simulink model "dvr_final"  (R2017b)
settings: Solver=ode45  StartTime=0.0  StopTime=1  RelTol=1e-3  EnableMultiTasking=on
undefined symbols (not defined in the file): D1, Delta, Ts
libraries: powerlib x28, powerlib_extras x19
settings Model: Creator=PRAVAT  LastModifiedBy=HP
settings DataIOCC: LimitDataPoints=on  SaveFormat=Array  SignalLoggingSaveFormat=ModelDataLogs
settings OptimizationCC: ExpressionDepthLimit=2147483647  LifeSpan=inf
settings DebuggingCC: UnderspecifiedInitializationDetection=Classic  MergeDetectMultiDrivingBlocksExec=none  SolverPrmCheckMsg=warning  FcnCallInpInsideContextMsg=warning  StateNameClashWarn=warning  StrictBusMsg=Warning  SFUnexpectedBacktrackingDiag=warning  SFNoUnconditionalDefaultTransitionDiag=warning  SFExecutionAtInitializationDiag=none
settings HardwareCC: ProdBitPerPointer=32  ProdBitPerSizeT=32  ProdBitPerPtrDiffT=32  ProdLargestAtomicFloat=None  ProdIntDivRoundTo=Undefined  ProdEndianess=Unspecified  ProdWordSize=32  ProdHWDeviceType=32-bit Generic
settings ModelReferenceCC: PropagateSignalLabelsOutOfModel=off
settings CodeAppCC: StateflowObjectComments=on
settings GRTTargetCC: TargetLangStandard=C89/C90 (ANSI)  CombineOutputUpdateFcns=off  GRTInterface=on
settings ConfigComp: CovMetricSettings=dw  CovHtmlReporting=on  CovSaveCumulativeToWorkspaceVar=on  CovSaveSingleToWorkspaceVar=on  CovExternalEMLEnable=off

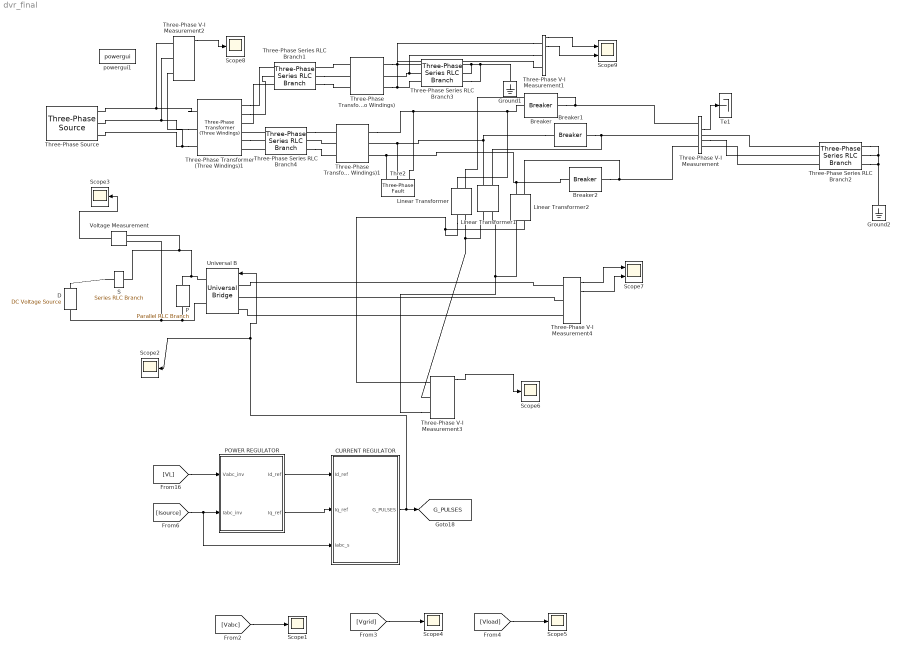
== system dvr_final ==
  Breaker : powerlib/Elements/Breaker  InitialState=1  SwitchingTimes=[0.4 0.6]  External=off  BreakerResistance=0.01  SnubberResistance=1e6  SnubberCapacitance=inf  Measurements=None  MoreParameters=off  NoBreakLoop=off
      settings: SourceProductName=Simscape Power Systems
  Breaker1 : powerlib/Elements/Breaker  InitialState=1  SwitchingTimes=[0.4 0.6]  External=off  BreakerResistance=0.01  SnubberResistance=1e6  SnubberCapacitance=inf  Measurements=None  MoreParameters=off  NoBreakLoop=off
      settings: SourceProductName=Simscape Power Systems
  Breaker2 : powerlib/Elements/Breaker  InitialState=1  SwitchingTimes=[0.4 0.6]  External=off  BreakerResistance=0.01  SnubberResistance=1e6  SnubberCapacitance=inf  Measurements=None  MoreParameters=off  NoBreakLoop=off
      settings: SourceProductName=Simscape Power Systems
  CURRENT REGULATOR : Subsystem
  D : powerlib/Electrical Sources/DC Voltage Source  Amplitude=5e3  Measurements=None
  Ground1 : powerlib/Elements/Ground  LConnTagsString=a
  Ground2 : powerlib/Elements/Ground  LConnTagsString=a
  Linear Transformer : powerlib/Elements/Linear Transformer  UNITS=pu  NominalPower=[ 250e6 50 ]  winding1="[11e3  0.002  0.08 ]"  winding2="[9e3  0.002  0.08 ]"  ThreeWindings=off  winding3=[ 60e3 0.005 0.02 ]  RmLm=[ 500 500 ]  Measurements=None  DataType=off
  Linear Transformer1 : powerlib/Elements/Linear Transformer  UNITS=pu  NominalPower=[ 250e6 50 ]  winding1="[11e3  0.002  0.08 ]"  winding2="[9e3  0.002  0.08 ]"  ThreeWindings=off  winding3=[ 60e3 0.005 0.02 ]  RmLm=[ 500 500 ]  Measurements=None  DataType=off
  Linear Transformer2 : powerlib/Elements/Linear Transformer  UNITS=pu  NominalPower=[ 250e6 50 ]  winding1="[11e3  0.002  0.08 ]"  winding2="[9e3  0.002  0.08 ]"  ThreeWindings=off  winding3=[ 60e3 0.005 0.02 ]  RmLm=[ 500 500 ]  Measurements=None  DataType=off
  P : powerlib/Elements/Parallel RLC Branch  LConnTagsString=a  RConnTagsString=__new0  BranchType=C  Resistance=[]  Inductance=[]  SetiL0=off  InitialCurrent=0  Capacitance=750e-6  Setx0=off  InitialVoltage=0  Measurements=Branch voltage and current
  POWER REGULATOR : Subsystem
  S : powerlib/Elements/Series RLC Branch  LConnTagsString=__new0  RConnTagsString=__new0  BranchType=R  Resistance=10  Inductance=1e-3  SetiL0=off  InitialCurrent=0  Capacitance=1e-6  Setx0=off  InitialVoltage=0  Measurements=None
  Scope{1..6,8} (7 alike) : Scope
  Scope7 : Scope  NumInputPorts=2
  Scope9 : Scope  NumInputPorts=2
  Te1 : Terminator
  Thre2 : powerlib/Elements/Three-Phase Fault  InitialStates=0  FaultA=on  FaultB=on  FaultC=on  GroundFault=on  SwitchTimes=[ 0.4 0.6]  External=off  SwitchStatus=NaN  FaultResistance=0.66  GroundResistance=0.4  SnubberResistance=1e6  SnubberCapacitance=inf  Measurements=None
  Three-Phase Series RLC Branch1 : powerlib/Elements/Three-Phase Series RLC Branch  LConnTagsString=A|B|C  RConnTagsString=A|B|C  BranchType=RL  Resistance=.05  Inductance=0.4806  Capacitance=1e-6  Measurements=None
  Three-Phase Series RLC Branch2 : powerlib/Elements/Three-Phase Series RLC Branch  LConnTagsString=A|B|C  RConnTagsString=A|B|C  BranchType=RL  Resistance=0.1  Inductance=.1926  Capacitance=1e-6  Measurements=Branch voltages
  Three-Phase Series RLC Branch3 : powerlib/Elements/Three-Phase Series RLC Branch  LConnTagsString=A|B|C  RConnTagsString=A|B|C  BranchType=R  Resistance=20  Inductance=1e-3  Capacitance=1e-6  Measurements=None
  Three-Phase Series RLC Branch4 : powerlib/Elements/Three-Phase Series RLC Branch  LConnTagsString=A|B|C  RConnTagsString=A|B|C  BranchType=RL  Resistance=0.001  Inductance=0.005  Capacitance=1e-6  Measurements=None
  Three-Phase Transformer (Three Windings)1 : powerlib/Elements/Three-Phase Transformer (Three Windings)  Winding1Connection=Yg  Winding2Connection=Delta (D1)  Winding3Connection=Delta (D1)  CoreType=Three single-phase transformers  SetSaturation=off  Hysteresis=off  DataFile='hysteresis'  SetInitialFlux=off  Measurements=None  UNITS=pu  NominalPower=[ 100e6 , 50 ]  Winding1=[13e3 , 0.002 , 0.08 ]  Winding2=[115e3 , 0.002 , 0.08 ]  Winding3=[115e3 , 0.002 , 0.08 ]  Rm=500  Lm=500  L0=0.5  Saturation=[ 0,0 ; 0.0024,1.2 ; 1.0,1.52 ]  InitialFluxes=[0.8 -0.8 0.7]  MoreParameters=off  BreakLoop=off  DataType=off  TransfoNumber=0
      settings: SourceProductName=Simscape Power Systems  SourceProductBaseCode=PS
  Three-Phase Transformer (Two Windings) : powerlib/Elements/Three-Phase Transformer (Two Windings)  Winding1Connection=Delta (D1)  Winding2Connection=Yg  CoreType=Three single-phase transformers  SetSaturation=off  Hysteresis=off  DataFile='hysteresis'  SetInitialFlux=off  Measurements=None  UNITS=pu  NominalPower=[ 250e6 , 50 ]  Winding1=[ 115e3 , 0.002 , 0.08 ]  Winding2=[ 11e3 , 0.002 , 0.08 ]  Rm=500  Lm=500  L0=0.5  Saturation=[ 0,0 ; 0.0024,1.2 ; 1.0,1.52 ]  InitialFluxes=[ 0.8 , -0.8 , 0.7 ]  MoreParameters=off  BreakLoop=off  DataType=off  TransfoNumber=0
  Three-Phase Transformer (Two Windings)1 : powerlib/Elements/Three-Phase Transformer (Two Windings)  Winding1Connection=Y  Winding2Connection=Delta (D1)  CoreType=Three single-phase transformers  SetSaturation=off  Hysteresis=off  DataFile='hysteresis'  SetInitialFlux=off  Measurements=None  UNITS=pu  NominalPower=[ 250e6 , 50 ]  Winding1=[ 115e3 , 0.002 , 0.08 ]  Winding2=[ 11e3 , 0.002 , 0.08 ]  Rm=500  Lm=500  L0=0.5  Saturation=[ 0,0 ; 0.0024,1.2 ; 1.0,1.52 ]  InitialFluxes=[ 0.8 , -0.8 , 0.7 ]  MoreParameters=off  BreakLoop=off  DataType=off  TransfoNumber=0
  Three-Phase V-I Measurement : powerlib/Measurements/Three-Phase V-I Measurement  VoltageMeasurement=phase-to-ground  SetLabelV=off  LabelV=Vabc  Vpu=on  VpuLL=off  CurrentMeasurement=yes  SetLabelI=off  LabelI=Iabc  Ipu=on  Pbase=100e6  Vbase=11e3  OutputType=Complex  PhasorSimulation=off  PSBequivalent=0
  Three-Phase V-I Measurement1 : powerlib/Measurements/Three-Phase V-I Measurement  VoltageMeasurement=phase-to-ground  SetLabelV=off  LabelV=Vabc  Vpu=on  VpuLL=off  CurrentMeasurement=yes  SetLabelI=off  LabelI=Iabc  Ipu=on  Pbase=100e6  Vbase=11e3  OutputType=Complex  PhasorSimulation=off  PSBequivalent=0
  Three-Phase V-I Measurement2 : powerlib/Measurements/Three-Phase V-I Measurement  VoltageMeasurement=phase-to-ground  SetLabelV=off  LabelV=Vabc  Vpu=on  VpuLL=off  CurrentMeasurement=yes  SetLabelI=off  LabelI=Iabc  Ipu=on  Pbase=100e6  Vbase=11e3  OutputType=Complex  PhasorSimulation=off  PSBequivalent=0
  Three-Phase V-I Measurement3 : powerlib/Measurements/Three-Phase V-I Measurement  VoltageMeasurement=phase-to-phase  SetLabelV=off  LabelV=Vabc  Vpu=on  VpuLL=off  CurrentMeasurement=yes  SetLabelI=off  LabelI=Iabc  Ipu=on  Pbase=100e6  Vbase=11e3  OutputType=Complex  PhasorSimulation=off  PSBequivalent=0
  Three-Phase V-I Measurement4 : powerlib/Measurements/Three-Phase V-I Measurement  VoltageMeasurement=phase-to-phase  SetLabelV=off  LabelV=Vabc  Vpu=on  VpuLL=off  CurrentMeasurement=yes  SetLabelI=off  LabelI=Iabc  Ipu=on  Pbase=100e6  Vbase=11e3  OutputType=Complex  PhasorSimulation=off  PSBequivalent=0
  Three-Phase Source : powerlib/Electrical Sources/Three-Phase Source  InternalConnection=Yg  VoltagePhases=off  Voltage=13e3  PhaseAngle=0  Voltage_phases=[25e3 25e3 25e3]/sqrt(3)  PhaseAngles_phases=[0 -120 +120]  Frequency=50  NonIdealSource=on  SpecifyImpedance=off  Resistance=0.1  Inductance=0  ShortCircuitLevel=100e6  BaseVoltage=25e3  XRratio=7  BusType=swing  Pref=10e3  Qref=0  Prefabc=[10e3, 10e3, 10e3]  Qrefabc=[0, 0, 0]  Qmin=-inf  Qmax=inf
  Universal B : powerlib/Power Electronics/Universal Bridge  Arms=3  SnubberResistance=1e5  SnubberCapacitance=inf  Device=IGBT / Diodes  Ron=1e-3  Lon=0  ForwardVoltages="[  0  0  ]"  ForwardVoltage=0  GTOparameters=[ 10e-6 , 20e-6 ]  IGBTparameters=[ 1e-6 , 2e-6 ]  Measurements=None  Measurements_2=None  converterType=Rectifier
      link override Uswitch: GotoTag=tp182559
  Voltage Measurement : powerlib/Measurements/Voltage Measurement  PhasorSimulation=off  OutputType=Complex  PSBequivalent=0
  powergui1 : powerlib/powergui  SimulationMode=Discrete  SampleTime=1e-5  frequency=60  Iterations=50  frequencyindice=50  Pbase=100e6  ErrMax=1e-4  UnitsV=kV  UnitsW=MW  buscounter=0  FunctionMessages=off  echomessages=off  EnableUseOfTLC=off  CurrentSourceSwitches=off  DisableSnubberDevices=off  DisableRonSwitches=off  DisableVfSwitches=off  DisplayEquations=off  SolverType=Tustin/Backward Euler (TBE)  Interpol=off  ExternalGateDelay=off  methode=off  Ts=0  x0status=blocks  SPID=off  SwTol=0  HookPort=off  RestoreLinks=warning  ResistiveCurrentMeasurement=off  Frange=[0:2:500]  Ylog=off  Xlog=on  ShowGrid=off  save=off  variable=ZData  structure=0  ZoomFFT=on  StartTime=0.0  cycles=1  DisplayStyle=1  fundamental=60  FreqAxis=off  MaxFrequency=1000  frequencyindicesteady=1  RmsSteady=1  display=off
  tag scope: G_PULSES=global
  wires:
  Voltage Measurement/1 -> Scope3/1
  Three-Phase V-I Measurement3/1 -> Scope6/1
  Three-Phase V-I Measurement4/1 -> Scope7/1
  CURRENT REGULATOR/1(G_PULSES) -> [G_PULSES], Universal B/1, Scope2/1
  POWER REGULATOR/1(Id_ref) -> CURRENT REGULATOR/1(Id_ref)
  POWER REGULATOR/2(Iq_ref) -> CURRENT REGULATOR/2(Iq_ref)
  [VL] -> POWER REGULATOR/1(Vabc_inv)
  [Isource] -> CURRENT REGULATOR/3(Iabc_s), POWER REGULATOR/2(Iabc_inv)
  [Vabc] -> Scope1/1
  [Vgrid] -> Scope4/1
  [Vload] -> Scope5/1
  Three-Phase V-I Measurement2/1 -> Scope8/1
  Three-Phase V-I Measurement/2 -> Te1/1
  Three-Phase V-I Measurement1/1 -> Scope9/1
  Three-Phase V-I Measurement1/2 -> Scope9/2
  Three-Phase V-I Measurement4/2 -> Scope7/2
  connections:
  P/LConn1 -- Universal B/RConn1 -- Voltage Measurement/LConn1 -- S/RConn1
  D/LConn1 -- Voltage Measurement/LConn2 -- Universal B/RConn2 -- P/RConn1
  Three-Phase V-I Measurement3/LConn1 -- Linear Transformer/RConn1 -- Linear Transformer2/RConn2
  Three-Phase V-I Measurement3/LConn2 -- Linear Transformer1/RConn1 -- Linear Transformer/RConn2
  Three-Phase V-I Measurement3/LConn3 -- Linear Transformer2/RConn1 -- Linear Transformer1/RConn2
  Three-Phase V-I Measurement4/LConn2 -- Universal B/LConn2
  Three-Phase V-I Measurement4/LConn1 -- Universal B/LConn1
  Three-Phase V-I Measurement4/LConn3 -- Universal B/LConn3
  S/LConn1 -- D/RConn1
  Three-Phase V-I Measurement1/LConn3 -- Three-Phase Transformer (Two Windings)/RConn3 -- Three-Phase Series RLC Branch3/LConn3
  Three-Phase Transformer (Three Windings)1/LConn2 -- Three-Phase Source/RConn2 -- Three-Phase V-I Measurement2/LConn2
  Breaker/RConn1 -- Linear Transformer/LConn2 -- Three-Phase V-I Measurement/LConn1
  Breaker1/LConn1 -- Linear Transformer1/LConn1 -- Thre2/LConn2 -- Three-Phase Transformer (Two Windings)1/RConn2
  Breaker/LConn1 -- Thre2/LConn1 -- Three-Phase Transformer (Two Windings)1/RConn1 -- Linear Transformer/LConn1
  Three-Phase Series RLC Branch2/RConn1 -- Ground2/LConn1 -- Three-Phase Series RLC Branch2/RConn3 -- Three-Phase Series RLC Branch2/RConn2
  Three-Phase Series RLC Branch3/RConn3 -- Three-Phase Series RLC Branch3/RConn2 -- Three-Phase Series RLC Branch3/RConn1 -- Ground1/LConn1
  Breaker1/RConn1 -- Linear Transformer1/LConn2 -- Three-Phase V-I Measurement/LConn2
  Three-Phase Transformer (Three Windings)1/LConn1 -- Three-Phase Source/RConn1 -- Three-Phase V-I Measurement2/LConn1
  Three-Phase Transformer (Three Windings)1/LConn3 -- Three-Phase Source/RConn3 -- Three-Phase V-I Measurement2/LConn3
  Three-Phase V-I Measurement1/LConn2 -- Three-Phase Series RLC Branch3/LConn2 -- Three-Phase Transformer (Two Windings)/RConn2
  Three-Phase V-I Measurement1/LConn1 -- Three-Phase Transformer (Two Windings)/RConn1 -- Three-Phase Series RLC Branch3/LConn1
  Breaker2/LConn1 -- Thre2/LConn3 -- Three-Phase Transformer (Two Windings)1/RConn3 -- Linear Transformer2/LConn1
  Breaker2/RConn1 -- Linear Transformer2/LConn2 -- Three-Phase V-I Measurement/LConn3
  Three-Phase V-I Measurement/RConn2 -- Three-Phase Series RLC Branch2/LConn2
  Three-Phase Series RLC Branch4/RConn3 -- Three-Phase Transformer (Two Windings)1/LConn3
  Three-Phase Series RLC Branch2/LConn3 -- Three-Phase V-I Measurement/RConn3
  Three-Phase Transformer (Three Windings)1/RConn1 -- Three-Phase Series RLC Branch1/LConn1
  Three-Phase Transformer (Two Windings)/LConn1 -- Three-Phase Series RLC Branch1/RConn1
  Three-Phase Transformer (Three Windings)1/RConn5 -- Three-Phase Series RLC Branch4/LConn2
  Three-Phase Transformer (Two Windings)1/LConn2 -- Three-Phase Series RLC Branch4/RConn2
  Three-Phase Series RLC Branch4/LConn3 -- Three-Phase Transformer (Three Windings)1/RConn6
  Three-Phase Series RLC Branch2/LConn1 -- Three-Phase V-I Measurement/RConn1
  Three-Phase Series RLC Branch1/LConn3 -- Three-Phase Transformer (Three Windings)1/RConn3
  Three-Phase Series RLC Branch4/RConn1 -- Three-Phase Transformer (Two Windings)1/LConn1
  Three-Phase Series RLC Branch4/LConn1 -- Three-Phase Transformer (Three Windings)1/RConn4
  Three-Phase Series RLC Branch1/RConn3 -- Three-Phase Transformer (Two Windings)/LConn3
  Three-Phase Transformer (Three Windings)1/RConn2 -- Three-Phase Series RLC Branch1/LConn2
  Three-Phase Series RLC Branch1/RConn2 -- Three-Phase Transformer (Two Windings)/LConn2

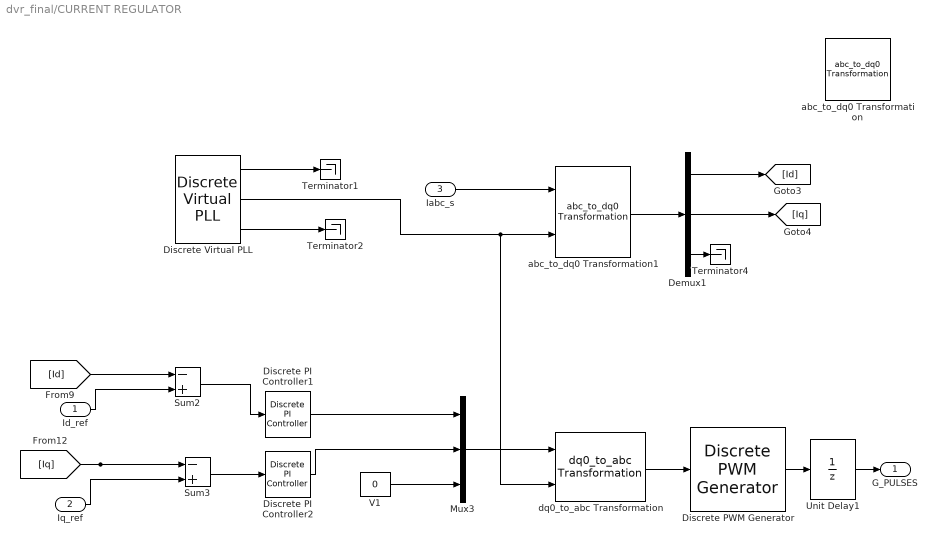
== system dvr_final/CURRENT REGULATOR ==
  Id_ref : Inport
  Iq_ref : Inport  Port=2
  Iabc_s : Inport  Port=3
  Demux1 : Demux  Outputs=3
  Discrete PI Controller1 : powerlib_extras/Discrete  Control Blocks/Discrete PI Controller  Kp=4  Ki=4000  Par_Limits=[1e6 -1e6]  Init=0  Ts=Ts
  Discrete PI Controller2 : powerlib_extras/Discrete  Control Blocks/Discrete PI Controller  Kp=4  Ki=4000  Par_Limits=[1e6 -1e6]  Init=0  Ts=Ts
  Discrete PWM Generator : powerlib_extras/Discrete  Control Blocks/Discrete PWM Generator  GeneratorMode="3-arm  bridge (6 pulses)"  Fc=8000  Ts=Ts  Internal=off  mIndex=0.8  Freq=60  Phase=0
  Discrete Virtual PLL : powerlib_extras/Discrete  Control Blocks/Discrete Virtual PLL  Freq=50  Phase=0  Ts=Ts
  Mux3 : Mux  Inputs=3
  Sum2 : Sum  Inputs=-+  SampleTime=Ts  SaturateOnIntegerOverflow=on  InputSameDT=on  OutDataTypeStr=Inherit: Same as first input
  Sum3 : Sum  Inputs=-+  SampleTime=Ts  SaturateOnIntegerOverflow=on  InputSameDT=on  OutDataTypeStr=Inherit: Same as first input
  Terminator1 : Terminator
  Terminator2 : Terminator
  Terminator4 : Terminator
  Unit Delay1 : UnitDelay  SampleTime=Ts
  V1 : Constant  Value=0  SampleTime=Ts
  abc_to_dq0 Transformation : powerlib_extras/Measurements/abc_to_dq0 Transformation
  abc_to_dq0 Transformation1 : powerlib_extras/Measurements/abc_to_dq0 Transformation
  dq0_to_abc Transformation : powerlib_extras/Measurements/dq0_to_abc Transformation
  G_PULSES : Outport
  wires:
  Demux1/3 -> Terminator4/1
  Demux1/2 -> [Iq]
  Demux1/1 -> [Id]
  abc_to_dq0 Transformation1/1 -> Demux1/1
  Iabc_s/1 -> abc_to_dq0 Transformation1/1
  Discrete Virtual PLL/3 -> Terminator2/1
  Discrete Virtual PLL/2 -> abc_to_dq0 Transformation1/2, dq0_to_abc Transformation/2
  Id_ref/1 -> Sum2/2
  Iq_ref/1 -> Sum3/2
  [Id] -> Sum2/1
  Sum2/1 -> Discrete PI Controller1/1
  Sum3/1 -> Discrete PI Controller2/1
  [Iq] -> Sum3/1
  Discrete PI Controller1/1 -> Mux3/1
  Discrete PI Controller2/1 -> Mux3/2
  V1/1 -> Mux3/3
  Discrete PWM Generator/1 -> Unit Delay1/1
  Unit Delay1/1 -> G_PULSES/1
  dq0_to_abc Transformation/1 -> Discrete PWM Generator/1
  Mux3/1 -> dq0_to_abc Transformation/1
  Discrete Virtual PLL/1 -> Terminator1/1

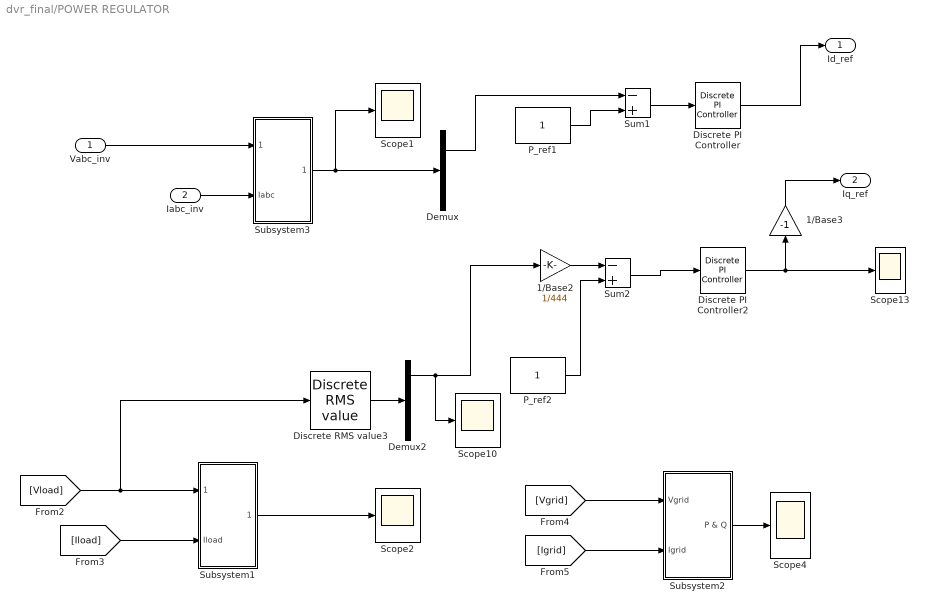
== system dvr_final/POWER REGULATOR ==
  Vabc_inv : Inport
  Iabc_inv : Inport  Port=2
  1/Base2 : Gain  Gain=1/444  SampleTime=Ts
  1/Base3 : Gain  Gain=-1  SampleTime=Ts
  Demux : Demux  Outputs=2
  Demux2 : Demux  Outputs=3
  Discrete PI Controller : powerlib_extras/Discrete  Control Blocks/Discrete PI Controller  Kp=0.4  Ki=3000  Par_Limits=[1e6 -1e6]  Init=0  Ts=Ts
  Discrete PI Controller2 : powerlib_extras/Discrete  Control Blocks/Discrete PI Controller  Kp=200  Ki=3800  Par_Limits=[1e6 -1e6]  Init=0  Ts=Ts
  Discrete RMS value3 : powerlib_extras/Discrete Measurements/Discrete  RMS value  Freq=50  Mag_Init=0  Ts=2e-6
  P_ref1 : Constant  SampleTime=Ts
  P_ref2 : Constant  SampleTime=Ts
  Scope{1..2,4,10,13} (5 alike) : Scope
  Subsystem1 : Subsystem
  Subsystem2 : Subsystem
  Subsystem3 : Subsystem
  Sum1 : Sum  Inputs=-+  SampleTime=Ts  SaturateOnIntegerOverflow=on  InputSameDT=on  OutDataTypeStr=Inherit: Same as first input
  Sum2 : Sum  Inputs=-+  SampleTime=Ts  SaturateOnIntegerOverflow=on  InputSameDT=on  OutDataTypeStr=Inherit: Same as first input
  Id_ref : Outport
  Iq_ref : Outport  Port=2
  wires:
  P_ref1/1 -> Sum1/2
  Sum1/1 -> Discrete PI Controller/1
  Discrete PI Controller/1 -> Id_ref/1
  Demux/1 -> Sum1/1
  Vabc_inv/1 -> Subsystem3/1(Vabc)
  Subsystem3/1(P & Q) -> Demux/1, Scope1/1
  Iabc_inv/1 -> Subsystem3/2(Iabc)
  [Vload] -> Subsystem1/1(Vload), Discrete RMS value3/1
  [Iload] -> Subsystem1/2(Iload)
  Subsystem1/1(P & Q) -> Scope2/1
  Subsystem2/1(P & Q) -> Scope4/1
  [Vgrid] -> Subsystem2/1(Vgrid)
  [Igrid] -> Subsystem2/2(Igrid)
  Demux2/1 -> 1/Base2/1, Scope10/1
  P_ref2/1 -> Sum2/2
  1/Base2/1 -> Sum2/1
  Sum2/1 -> Discrete PI Controller2/1
  Discrete PI Controller2/1 -> 1/Base3/1, Scope13/1
  Discrete RMS value3/1 -> Demux2/1
  1/Base3/1 -> Iq_ref/1

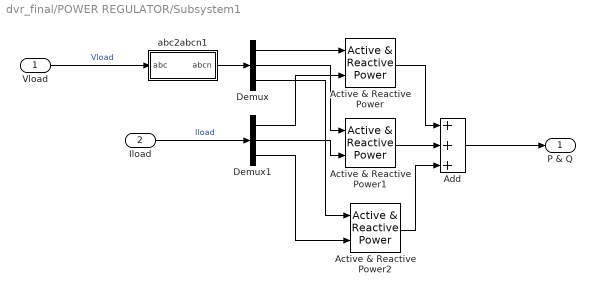
== system dvr_final/POWER REGULATOR/Subsystem1 ==
  Vload : Inport
  Iload : Inport  RequirementInfo={} %GIDa_a0c317ec_178d_488c_8ae0_b396030d6192  Port=2
  Active & Reactive Power : powerlib_extras/Measurements/Active & Reactive Power  f1=50
  Active & Reactive Power1 : powerlib_extras/Measurements/Active & Reactive Power  f1=50
  Active & Reactive Power2 : powerlib_extras/Measurements/Active & Reactive Power  f1=50
  Add : Sum  Inputs=+++
  Demux : Demux  Outputs=3
  Demux1 : Demux  Outputs=3
  abc2abcn1 : Subsystem
  P & Q : Outport
  wires:
  abc2abcn1/1(abcn) -> Demux/1
  Demux/1 -> Active & Reactive Power/1
  Demux1/1 -> Active & Reactive Power/2
  Demux/2 -> Active & Reactive Power1/1
  Demux/3 -> Active & Reactive Power2/1
  Demux1/2 -> Active & Reactive Power1/2
  Demux1/3 -> Active & Reactive Power2/2
  Active & Reactive Power/1 -> Add/1
  Active & Reactive Power1/1 -> Add/2
  Active & Reactive Power2/1 -> Add/3
  Add/1 -> P & Q/1
  Vload/1 -> abc2abcn1/1(abc)  "Vload"
  Iload/1 -> Demux1/1  "Iload"

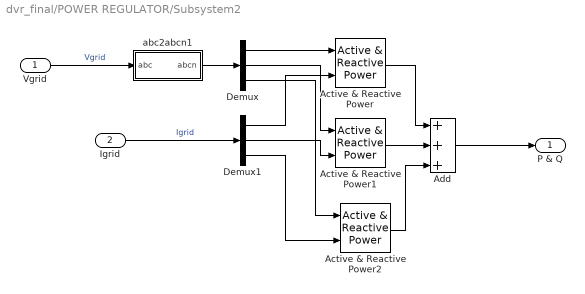
== system dvr_final/POWER REGULATOR/Subsystem2 ==
  Vgrid : Inport
  Igrid : Inport  RequirementInfo={} %GIDa_a0c317ec_178d_488c_8ae0_b396030d6192  Port=2
  Active & Reactive Power : powerlib_extras/Measurements/Active & Reactive Power  f1=50
  Active & Reactive Power1 : powerlib_extras/Measurements/Active & Reactive Power  f1=50
  Active & Reactive Power2 : powerlib_extras/Measurements/Active & Reactive Power  f1=50
  Add : Sum  Inputs=+++
  Demux : Demux  Outputs=3
  Demux1 : Demux  Outputs=3
  abc2abcn1 : Subsystem
  P & Q : Outport
  wires:
  abc2abcn1/1(abcn) -> Demux/1
  Demux/1 -> Active & Reactive Power/1
  Demux1/1 -> Active & Reactive Power/2
  Demux/2 -> Active & Reactive Power1/1
  Demux/3 -> Active & Reactive Power2/1
  Demux1/2 -> Active & Reactive Power1/2
  Demux1/3 -> Active & Reactive Power2/2
  Active & Reactive Power/1 -> Add/1
  Active & Reactive Power1/1 -> Add/2
  Active & Reactive Power2/1 -> Add/3
  Add/1 -> P & Q/1
  Vgrid/1 -> abc2abcn1/1(abc)  "Vgrid"
  Igrid/1 -> Demux1/1  "Igrid"

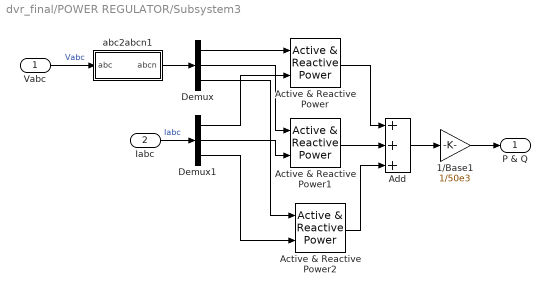
== system dvr_final/POWER REGULATOR/Subsystem3 ==
  Vabc : Inport
  Iabc : Inport  RequirementInfo={} %GIDa_a0c317ec_178d_488c_8ae0_b396030d6192  Port=2
  1/Base1 : Gain  Gain=1/50e3  SampleTime=Ts
  Active & Reactive Power : powerlib_extras/Measurements/Active & Reactive Power  f1=50
  Active & Reactive Power1 : powerlib_extras/Measurements/Active & Reactive Power  f1=50
  Active & Reactive Power2 : powerlib_extras/Measurements/Active & Reactive Power  f1=50
  Add : Sum  Inputs=+++
  Demux : Demux  Outputs=3
  Demux1 : Demux  Outputs=3
  abc2abcn1 : Subsystem
  P & Q : Outport
  wires:
  abc2abcn1/1(abcn) -> Demux/1
  Demux/1 -> Active & Reactive Power/1
  Demux1/1 -> Active & Reactive Power/2
  Demux/2 -> Active & Reactive Power1/1
  Demux/3 -> Active & Reactive Power2/1
  Demux1/2 -> Active & Reactive Power1/2
  Demux1/3 -> Active & Reactive Power2/2
  Active & Reactive Power/1 -> Add/1
  Active & Reactive Power1/1 -> Add/2
  Active & Reactive Power2/1 -> Add/3
  Vabc/1 -> abc2abcn1/1(abc)  "Vabc"
  Iabc/1 -> Demux1/1  "Iabc"
  Add/1 -> 1/Base1/1
  1/Base1/1 -> P & Q/1

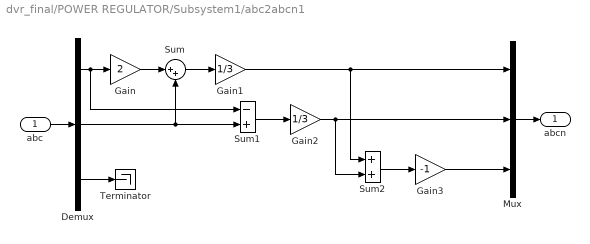
== system dvr_final/POWER REGULATOR/Subsystem1/abc2abcn1 ==
  abc : Inport
  Demux : Demux  Outputs=3
  Gain : Gain  Gain=2
  Gain1 : Gain  Gain=1/3
  Gain2 : Gain  Gain=1/3
  Gain3 : Gain  Gain=-1
  Mux : Mux  Inputs=3
  Sum : Sum  Inputs=|++
  Sum1 : Sum  Inputs=-+
  Sum2 : Sum
  Terminator : Terminator
  abcn : Outport
  wires:
  abc/1 -> Demux/1
  Mux/1 -> abcn/1
  Gain3/1 -> Mux/3
  Sum2/1 -> Gain3/1
  Gain2/1 -> Mux/2, Sum2/2
  Gain1/1 -> Mux/1, Sum2/1
  Sum1/1 -> Gain2/1
  Demux/3 -> Terminator/1
  Sum/1 -> Gain1/1
  Demux/2 -> Sum1/2, Sum/2
  Gain/1 -> Sum/1
  Demux/1 -> Sum1/1, Gain/1

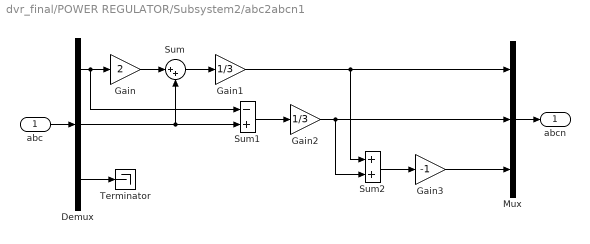
== system dvr_final/POWER REGULATOR/Subsystem2/abc2abcn1 ==
  abc : Inport
  Demux : Demux  Outputs=3
  Gain : Gain  Gain=2
  Gain1 : Gain  Gain=1/3
  Gain2 : Gain  Gain=1/3
  Gain3 : Gain  Gain=-1
  Mux : Mux  Inputs=3
  Sum : Sum  Inputs=|++
  Sum1 : Sum  Inputs=-+
  Sum2 : Sum
  Terminator : Terminator
  abcn : Outport
  wires:
  abc/1 -> Demux/1
  Mux/1 -> abcn/1
  Gain3/1 -> Mux/3
  Sum2/1 -> Gain3/1
  Gain2/1 -> Mux/2, Sum2/2
  Gain1/1 -> Mux/1, Sum2/1
  Sum1/1 -> Gain2/1
  Demux/3 -> Terminator/1
  Sum/1 -> Gain1/1
  Demux/2 -> Sum1/2, Sum/2
  Gain/1 -> Sum/1
  Demux/1 -> Sum1/1, Gain/1

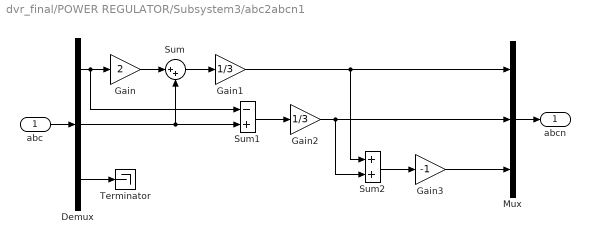
== system dvr_final/POWER REGULATOR/Subsystem3/abc2abcn1 ==
  abc : Inport
  Demux : Demux  Outputs=3
  Gain : Gain  Gain=2
  Gain1 : Gain  Gain=1/3
  Gain2 : Gain  Gain=1/3
  Gain3 : Gain  Gain=-1
  Mux : Mux  Inputs=3
  Sum : Sum  Inputs=|++
  Sum1 : Sum  Inputs=-+
  Sum2 : Sum
  Terminator : Terminator
  abcn : Outport
  wires:
  abc/1 -> Demux/1
  Mux/1 -> abcn/1
  Gain3/1 -> Mux/3
  Sum2/1 -> Gain3/1
  Gain2/1 -> Mux/2, Sum2/2
  Gain1/1 -> Mux/1, Sum2/1
  Sum1/1 -> Gain2/1
  Demux/3 -> Terminator/1
  Sum/1 -> Gain1/1
  Demux/2 -> Sum1/2, Sum/2
  Gain/1 -> Sum/1
  Demux/1 -> Sum1/1, Gain/1
